simulink library "RadarImagingAndPositioning"  (R2018a)
settings: Solver=VariableStepAuto  StartTime=0.0  StopTime=10.0  RelTol=1e-3
undefined symbols (not defined in the file): fft2, gather, get, gpuArray, Time, us
libraries: dspobslib x8, dspstat3 x3, visionsinks x2, dspfdesign x2, commsdrhw_v2 x1, dspbuff3 x1, visiontransforms x1, dspsigops x1
settings Model: Creator=Sky  LastModifiedBy=Sky

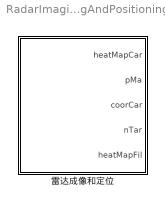
== system RadarImagingAndPositioning ==
  雷达成像和定位 : Subsystem  mask{yLoDownFac=2, nCyclePF=1, lFftAng=128, lFftDis=256, yMi=1, yMa=10, nTarMa=5, nFavr=40, pBackThres=0.0125, lWfil=3, pRelaThres=10, doSaveParam=on, decimInterp=100, rxBits=logical(dec2bin(0:11)-48), txBits=logical(dec2bin(0:3)-48), rxCoor=single([linspace(-0.053*(12/2-0.5),0.053*(12/2-0.5),12)',zeros(12,2)]), txCoor=single([zeros(4,2),linspace(-0.138-0.053*3,-0.138,4)']), dCa=4.65+0.5, fRamp=2000, fCen=3.2e9, fBw=1e9, tPul=0.0245e-3, tPulF=0.050e-3, trEdge=0, trThres=0}
      mask prompts: yLoDownFac "yLo downsample factor"; nCyclePF "cycles per frame (average time)"; lFftAng "angle FFT length"; lFftDis "dis FFT length"; yMi "y min"; yMa "y max"; nTarMa "targets number max"; nFavr "average frames"; pBackThres "background power threshold"; lWfil "filter window width"; pRelaThres "targets relative threshold"; doSaveParam "save parameters to workspace"; decimInterp "decimation factor"; rxBits "Rx bits"; txBits "Tx bits"; rxCoor "rx coordinates"; txCoor "tx coordinates"; dCa "cable length"; fRamp "ramp frequency"; fCen "center frequency"; fBw "bandwidth"; tPul "pulse width"; tPulF "first pulse width"; trEdge "triger edge"; trThres "triger threshold"
      mask help:
      | 雷达成像和定位模块。包含雷达成像和目标检测的主要算法。参数中USRP、Hardware、Ramp Parameters板块下的参数均与硬件有关，若有调整需求，请联系作者。
      |
      | 端口说明：
      | - heatMapCar：笛卡尔坐标系的雷达图像，经过对比度调整可以直接显示。
      | - pMa：雷达图像最大功率值。参考该值设置Targeting Parameters板块下的background power threshold参数，保证无人状态下的pMa小于参数background power threshold。算法原理：当pMa < background power threshold时判定区域内没有目标，此时端口nTar输出的值为0。
      | - coorTar：n行2列的矩阵，n个目标的坐标，单位（m）。第1列为x坐标，第2列为y坐标。前nTar个坐标为有效坐标。
      | - nTar：目标的个数。
      | - heatMapFil：滤波后的图像。算法原理：由于帧平均后的图像一个目标可能引起多个峰值，因此对图像进行一次以filter window width为正方形窗口宽度的中值滤波和均值滤波。增加filter window width使滤波后的图像更加平滑，减少一个目标检测到多个点的可能，同时会增加运算量。该端口用作参考以对filter window width进行修改。
      |
      | 参数说明：参数中Preprocess、FFT、Imaging、Targeting Parameters板块下的参数影响了运算量和目标检测效果。
      | - Preprocess Parameters：
      |     - yLo downsample factor：中频信号软件降采样系数。增大此值以减小运算量，同时减小距离测量范围。
      |     - cycles per frame（average time）：每帧包含的天线扫描周期。算法原理：将多个周期的中频信号平均，合并为一帧。增大此值以减小运算量，同时降低帧率。
      | - FFT Parameters：
      |     - angle FFT length：角度方向的FFT长度，设置为2的幂次方以使用更快的FFT算法。
      |     - dis FFT length：距离方向的FFT长度，设置为2的幂次方以使用更快的FFT算法。
      | - Imaging Parameters：
      |     - y min（max）：距离方向（y 方向）的坐标范围，直接影响雷达图像的行数和坐标序列ys，单位（m）。算法原理：两个参数会将2DFFT后的矩阵在距离方向（y方向）上作截取，如果dis FFT length参数设置的FFT长度达不到y max参数要求的FFT长度，会自动截取到dis FFT length所能计算到的最远距离，此ys表示的坐标序列不再以y max为最大值。
      | - Targeting Parameters：
      |     - target number max：最大跟踪目标数量。
      |     - average frames：滑动均值滤波的窗口宽度。算法原理：多径效应对成像造成的影响一般呈现出瞬时性，如果通过滑动均值滤波的方法平均多帧雷达图像，可以大大减弱多径效应的影响。同时均值滤波会带来与窗口长度相同的延迟。
      |     - background power threshold：背景功率阈值。参考pMa端口输出的功率设置Targeting Parameters板块下的background power threshold参数，保证无人状态下的pMa小于参数background power threshold。算法原理：当pMa < background power threshold时判定区域内没有目标，此时端口nTar输出的值为0。
      |     - filter window width：图像滤波的窗口宽度，设置为3以上的奇数（如3、5、7……）。算法原理：由于帧平均后的图像一个目标可能引起多个峰值，因此对图像进行一次以filter window width为正方形窗口宽度的中值滤波和均值滤波。增加此值使滤波后的图像更加平滑，减少一个目标检测到多个点的可能，同时会增加运算量。可以参考端口heaMapFil输出的滤波后的图像对该值进行修改。
      |     - targets relative threshold：目标功率相对与背景噪声功率比值的阈值。算法原理：以背景噪声平均值的targets relative threshold倍作为阈值对图像进行分割，高于此阈值的像素认为有目标存在。
      mask init:
      | if doSaveParam
      |     evalin('base','clear');
      | end
      | 
      | % 天线和斜坡参数
      | nRx=size(rxBits,1);
      | nTx=size(txBits,1);
      | lFraw=100e6/decimInterp/fRamp*nRx*nTx*nCyclePF;
      | fSraw=100e6/decimInterp;
      | fSdown=fSraw/yLoDownFac;
      | fF=fSraw/lFraw;
      | lRampRaw=fSraw/fRamp;%length ramp raw
      | lRampDown=lRampRaw/yLoDownFac;%length ramp downsample
      | nPul=size(rxBits,2)+size(txBits,2)+1;
      | lPul=fSraw*tPul;%length pulse
      | lPulF=fSraw*tPulF;%length pulse first
      | 
      | dLambda=3e8/fCen;
      | fPm=fBw*fRamp/3e8;%frequency per meter
      | fD=fSdown/lFftDis;%frequency delta
      | fs=single(linspace(0,fSraw/yLoDownFac/2-fD,floor(lFftDis/2)));
      | ds=fs/fPm;
      | 
      | angMax=asind(dLambda/2/abs(rxCoor(1,1)-rxCoor(2,1)));
      | angs=single(linspace(-angMax,angMax,lFftAng));
      | 
      | % 排除线缆长度，截取有效距离
      | dsVal=(ds(ds>=dCa)-dCa)/2;
      | isDval=single(find(dsVal>=yMi & dsVal<=yMa));
      | dsVal=dsVal(isDval);
      | isDval=isDval+find(ds>=dCa,1)-1;
      | 
      | % 一个斜坡内的时间
      | tsRampDown=single((0:lRampRaw/yLoDownFac-1)/fSraw*yLoDownFac);
      | isDown=yLoDownFac:yLoDownFac:lFraw;
      | 
      | % 极坐标转换后的xy坐标
      | ys=dsVal;
      | xsMax=sind(max(abs(angs)))*max(abs(dsVal));
      | xs=linspace(-xsMax,xsMax,length(angs));
      | [xss,yss]=meshgrid(xs,ys);
      | 
      | % 极坐标转换矩阵
      | dsPo2Car=sqrt(xss.^2+yss.^2);
      | angsPo2Car=atand(xss./yss);
      | angsPo2Car(isnan(angsPo2Car))=0;
      | 
      | % 计算衰减因子
      | facD=repmat((dsVal.^4)',1,length(angs));
      | 
      | % 保存参数到工作空间base
      | if doSaveParam
      |     % mask变量
      |     assignin('base','rxBits',rxBits);
      |     assignin('base','txBits',txBits);
      |     assignin('base','rxCoor',rxCoor);
      |     assignin('base','txCoor',txCoor);
      |     assignin('base','dCa',dCa);
      |     assignin('base','fRamp',fRamp);
      |     assignin('base','fCen',fCen);
      |     assignin('base','fBw',fBw);
      |     assignin('base','tPul',tPul);
      |     assignin('base','yLoDownFac',yLoDownFac);
      |     assignin('base','nCyclePF',nCyclePF);
      |     assignin('base','lFftAng',lFftAng);
      |     assignin('base','lFftDis',lFftDis);
      | 
      |     assignin('base','yMi',yMi);
      |     assignin('base','yMa',yMa);
      |     
      |     % 全局变量
      |     assignin('base','nRx',nRx);
      |     assignin('base','nTx',nTx);
      |     assignin('base','lFraw',lFraw);
      |     assignin('base','fF',fF);
      |     assignin('base','fSraw',fSraw);
      |     assignin('base','fSdown',fSdown);
      |     assignin('base','fPm',fPm);
      |     assignin('base','lRampRaw',lRampRaw);
      |     assignin('base','lRampDown',lRampDown);
      |     assignin('base','dLambda',dLambda);
      |     assignin('base','ds',ds);
      |     assignin('base','angs',angs);
      |     assignin('base','dsVal',dsVal);
      |     assignin('base','isDval',isDval);
      |     assignin('base','tsRamp',tsRampDown);
      |     assignin('base','xs',xs);
      |     assignin('base','ys',ys);
      |     assignin('base','xss',xss);
      |     assignin('base','yss',yss);
      |     assignin('base','facD',facD);
      | end
      mask TypeOptions decimInterp: SDRu Receiver/decimInterp
      mask DialogControl Container16 Prompt: 软件相关
      mask DialogControl preParams Prompt: Preprocess Parameters
      mask DialogControl fftParams Prompt: FFT Parameters
      mask DialogControl imagParams Prompt: Imaging Parameters
      mask DialogControl tarParams Prompt: Targeting Parameters
      mask DialogControl tabHardwareRelated Prompt: 硬件相关
      mask DialogControl simParam Prompt: sim parameters
      mask DialogControl USRPparams Prompt: USRP Parameters
      mask DialogControl hwParams Prompt: Hardware Parameters
      mask DialogControl rampParams Prompt: Ramp Parameters
      mask DialogControl tabDescription Prompt: 说明

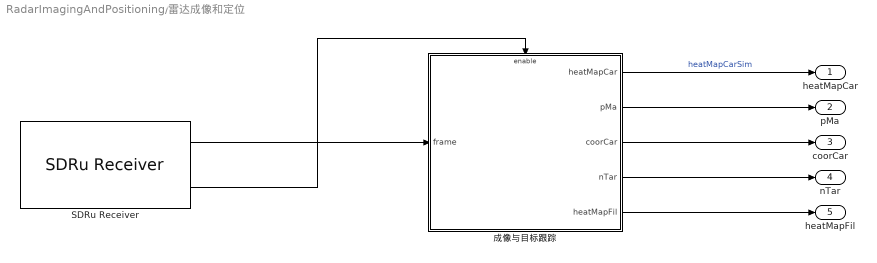
== system RadarImagingAndPositioning/雷达成像和定位 ==
  SDRu Receiver : commsdrhw_v2/SDRu Receiver  SourceLibraryInfo="This block requires <a href=\"http://www.mathworks.com/hardware-support/usrp.html\">Communications System Toolbox Support Package for USRP Radio</a>"  rxtx=rx  initializeIPAddress=0  devMap=0  USRP2_IP=192.168.10.6  USRP_IP_X300=192.168.10.2  USRP_IP_X310=192.168.10.2  USRP_serialNumB200=No devices found  USRP_serialNumB210=No devices found  platform=N200/N210/USRP2  prevPlatform=N200/N210/USRP2  lastIPAddressPopup=192.168.10.2  USRP_ID=192.168.10.6  LastIPAddress=192.168.10.2  ChannelMapping=1  centerFrequencySrc=Dialog  centerFrequency=0  loOffsetSrc=Dialog  loOffset=0  gainSrc=Dialog  gain=0  PPSSource=Internal  clockSource=Internal  masterClkRateParam=100e6  masterClkRateB200=32e6  masterClkRateB210=32e6  masterClkRateX300=200e6  masterClkRateX310=200e6  masterClkRate=100e6  decimInterpSrc=Dialog  decimInterp=decimInterp  USRP2_IP_NUM=[49 57 50 46 49 54 56 46 49 48 46 54]  TransportDataType=int16  overrunUnderrunPort=off  sampleTime=decimInterp/100e6  outputDatatype=single  frameLength=lFraw  HOST_DATA_PORT=0  HOST_CONTROL_PORT=0  USRP2_DATA_PORT=0  USRP2_CONTROL_PORT=0  bufferMode=Continuous streaming  EnableBurstMode=off  NumFramesInBurst=10000
      settings: SourceProductName=Communications System Toolbox Support Package for USRP(R) Radio  SourceProductBaseCode=USRP
  成像与目标跟踪 : Subsystem
  heatMapCar : Outport
  pMa : Outport  Port=2
  coorCar : Outport  Port=3
  nTar : Outport  Port=4
  heatMapFil : Outport  Port=5
  wires:
  SDRu Receiver/2 -> 成像与目标跟踪/Enable
  SDRu Receiver/1 -> 成像与目标跟踪/1(frame)
  成像与目标跟踪/1(heatMapCar) -> heatMapCar/1  "heatMapCarSim"
  成像与目标跟踪/4(nTar) -> nTar/1
  成像与目标跟踪/2(pMa) -> pMa/1
  成像与目标跟踪/3(coorCar) -> coorCar/1
  成像与目标跟踪/5(heatMapFil) -> heatMapFil/1

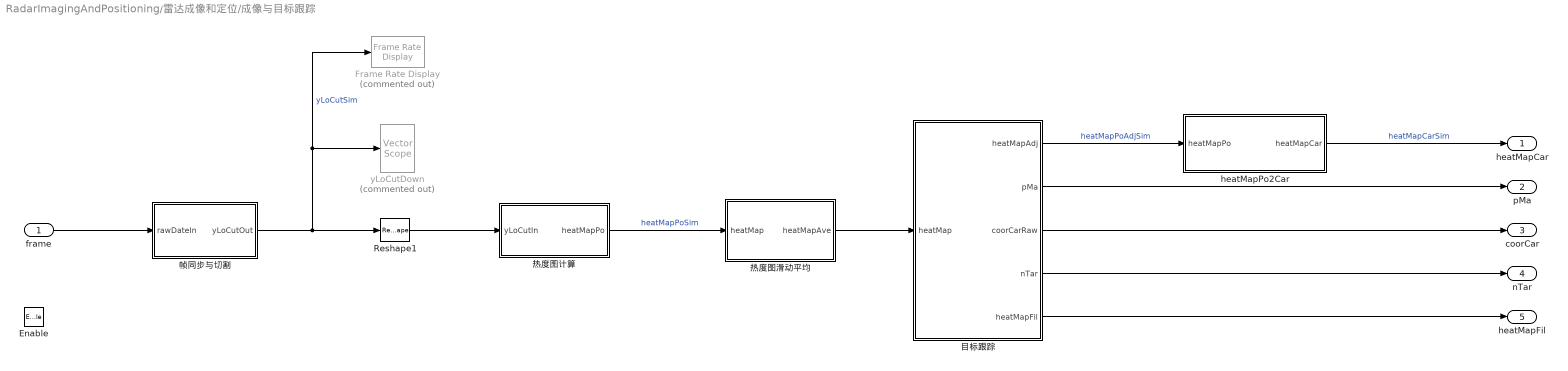
== system RadarImagingAndPositioning/雷达成像和定位/成像与目标跟踪 ==
  frame : Inport
  Enable : EnablePort  PropagateVarSize=During execution
  Frame Rate Display : visionsinks/Frame Rate Display  Commented=on  UpdateRate=10
      settings: SourceProductName=Computer Vision System Toolbox  SourceProductBaseCode=VP
  Reshape1 : Reshape  OutputDimensionality=Customize  OutputDimensions=[lRampDown,nRx,nTx]
  heatMapPo2Car : MATLAB Function  TreatAsAtomicUnit=on
  yLoCutDown : dspobslib/Vector Scope  Commented=on  ScopeProperties=on  Domain=User-defined  HorizSpan=1  DisplayProperties=off  AxisGrid=on  Memory=off  FrameNumber=on  AxisLegend=off  AxisZoom=off  OpenScopeAtSimStart=on  OpenScopeImmediately=off  FigPos=get(0,'defaultfigureposition')  AxisProperties=off  XUnits=Hertz  XRange=[0...Fs/2]  InheritXIncr=off  XIncr=1e6/fSdown  XLabel=Time(us)  XLimit=Auto  XMin=0  XMax=1  XStart=0  YUnits=dB  YLabel=Amplitude  LineProperties=off  LineColors=[1 0 0]|[0 1 0]|[0 0 1]  XAxisParamsVer=6.9
      settings: SourceProductName=DSP System Toolbox  SourceProductBaseCode=DS  YMin=-0.3  YMax=0.3
  帧同步与切割 : Subsystem
  热度图滑动平均 : Subsystem
  热度图计算 : Subsystem
  目标跟踪 : Subsystem
  heatMapCar : Outport
  pMa : Outport  Port=2
  coorCar : Outport  Port=3
  nTar : Outport  Port=4
  heatMapFil : Outport  Port=5
  wires:
  目标跟踪/1(heatMapAdj) -> heatMapPo2Car/1(heatMapPo)  "heatMapPoAdjSim"
  热度图滑动平均/1(heatMapAve) -> 目标跟踪/1(heatMap)
  热度图计算/1(heatMapPo) -> 热度图滑动平均/1(heatMap)  "heatMapPoSim"
  目标跟踪/3(coorCarRaw) -> coorCar/1
  帧同步与切割/1(yLoCutOut) -> Reshape1/1, Frame Rate Display/1, yLoCutDown/1  "yLoCutSim"
  frame/1 -> 帧同步与切割/1(rawDateIn)
  Reshape1/1 -> 热度图计算/1(yLoCutIn)
  目标跟踪/2(pMa) -> pMa/1
  目标跟踪/4(nTar) -> nTar/1
  heatMapPo2Car/1(heatMapCar) -> heatMapCar/1  "heatMapCarSim"
  目标跟踪/5(heatMapFil) -> heatMapFil/1

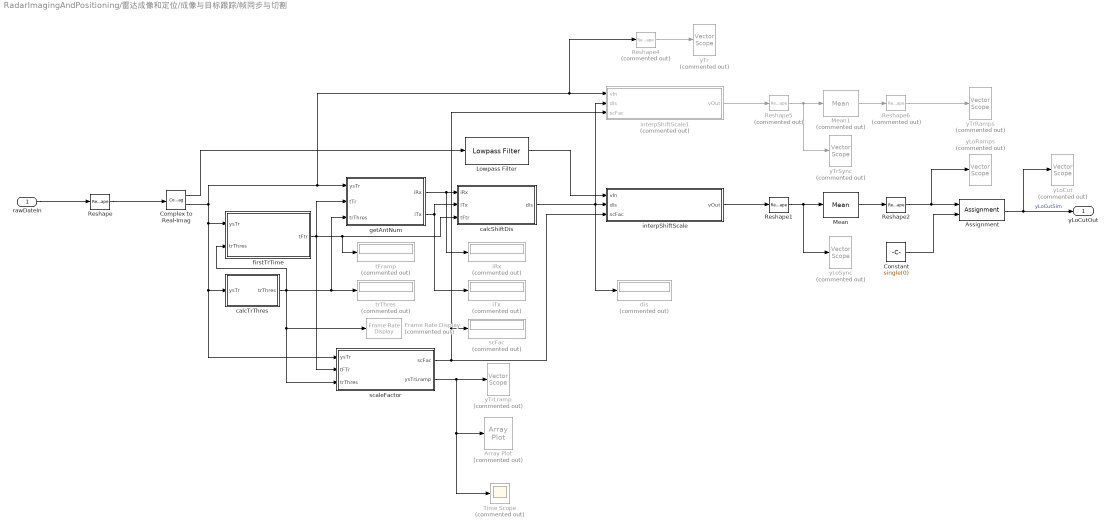
== system RadarImagingAndPositioning/雷达成像和定位/成像与目标跟踪/帧同步与切割 ==
  rawDateIn : Inport
  Array Plot : ArrayPlot  Commented=on
  Assignment : Assignment  NumberOfDimensions=2  DiagnosticForDimensions=Warning  IndexOptions=Index vector (dialog),Assign all  Indices=[1:ceil(2e-5*fSdown),lRampDown-ceil(2e-5*fSdown):lRampDown],1  OutputSizes=1,1
  Complex to Real-Imag : ComplexToRealImag
  Constant : Constant  Value=single(0)
  Frame Rate Display : visionsinks/Frame Rate Display  Commented=on  UpdateRate=10
      settings: SourceProductName=Computer Vision System Toolbox  SourceProductBaseCode=VP
  Lowpass Filter : dspfdesign/Lowpass Filter  FilterType=FIR  DesignForMinimumOrder=on  FilterOrder=20  PassbandFrequency=0.3*fSdown  StopbandFrequency=min(0.7*fSdown,0.5*fSraw)  PassbandRipple=0.1  StopbandAttenuation=50  InheritSampleRate=off  SampleRate=fSraw  SimulateUsing=Interpreted execution  roundingMode=Floor  coeffsDataTypeStr=fixdt(1,16)
  Mean : dspstat3/Mean  run=off  InputProcessing=Columns as channels (frame based)  reset_popup=None  directionMode=Each row  dimension=1  roiEnable=off  roiType=Rectangles  roiPortion=Entire ROI  roiOutput=Individual statistics for each ROI  roiFlag=off  roundingMode=Floor  overflowMode=off  outputDataTypeStr=Inherit: Same as accumulator  outputMin=[]  outputMax=[]  outputLastDataTypeStr=Inherit: Same as accumulator
  Mean1 : dspstat3/Mean  Commented=on  run=off  InputProcessing=Columns as channels (frame based)  reset_popup=None  directionMode=Each row  dimension=1  roiEnable=off  roiType=Rectangles  roiPortion=Entire ROI  roiOutput=Individual statistics for each ROI  roiFlag=off  roundingMode=Floor  overflowMode=off  outputDataTypeStr=Inherit: Same as accumulator  outputMin=[]  outputMax=[]  outputLastDataTypeStr=Inherit: Same as accumulator
  Reshape : Reshape  OutputDimensionality=Column vector (2-D)
  Reshape1 : Reshape  OutputDimensionality=Customize  OutputDimensions=[lRampDown*nRx*nTx,nCyclePF]
  Reshape2 : Reshape  OutputDimensionality=Customize  OutputDimensions=[lRampDown,nRx*nTx]
  Reshape4 : Reshape  Commented=on  OutputDimensionality=Column vector (2-D)
  Reshape5 : Reshape  Commented=on  OutputDimensionality=Customize  OutputDimensions=[lRampDown*nRx*nTx,nCyclePF]
  Reshape6 : Reshape  Commented=on  OutputDimensionality=Customize  OutputDimensions=[lRampDown,nRx*nTx]
  Time Scope : Scope  Commented=on
  calcShiftDis : MATLAB Function  TreatAsAtomicUnit=on
  calcTrThres : MATLAB Function  TreatAsAtomicUnit=on
  dis : Display  Commented=on
  firstTrTime : MATLAB Function  TreatAsAtomicUnit=on
  getAntNum : MATLAB Function  TreatAsAtomicUnit=on
  iRx : Display  Commented=on
  iTx : Display  Commented=on
  interpShiftScale : MATLAB Function  TreatAsAtomicUnit=on
  interpShiftScale1 : MATLAB Function  Commented=on  TreatAsAtomicUnit=on
  scFac : Display  Commented=on
  scaleFactor : MATLAB Function  TreatAsAtomicUnit=on
  tFramp : Display  Commented=on
  trThres : Display  Commented=on
  yLoCut : dspobslib/Vector Scope  Commented=on  ScopeProperties=on  Domain=User-defined  HorizSpan=1  DisplayProperties=off  AxisGrid=on  Memory=off  FrameNumber=on  AxisLegend=off  AxisZoom=off  OpenScopeAtSimStart=on  OpenScopeImmediately=off  FigPos=get(0,'defaultfigureposition')  AxisProperties=off  XUnits=Hertz  XRange=[0...Fs/2]  InheritXIncr=off  XIncr=1e6/fSdown  XLabel=Time(us)  XLimit=Auto  XMin=0  XMax=1  XStart=0  YUnits=dB  YLabel=Amplitude  LineProperties=off  LineColors=[1 0 0]|[0 1 0]|[0 0 1]  XAxisParamsVer=6.9
      settings: SourceProductName=DSP System Toolbox  SourceProductBaseCode=DS  YMin=-0.3  YMax=0.3
  yLoRamps : dspobslib/Vector Scope  Commented=on  ScopeProperties=on  Domain=User-defined  HorizSpan=1  DisplayProperties=off  AxisGrid=on  Memory=off  FrameNumber=on  AxisLegend=off  AxisZoom=off  OpenScopeAtSimStart=on  OpenScopeImmediately=off  FigPos=get(0,'defaultfigureposition')  AxisProperties=off  XUnits=Hertz  XRange=[0...Fs/2]  InheritXIncr=off  XIncr=1e6/fSdown  XLabel=Time(us)  XLimit=Auto  XMin=0  XMax=1  XStart=0  YUnits=dB  YLabel=Amplitude  LineProperties=off  LineColors=[1 0 0]|[0 1 0]|[0 0 1]  XAxisParamsVer=6.9
      settings: SourceProductName=DSP System Toolbox  SourceProductBaseCode=DS  YMin=-0.3  YMax=0.3
  yLoSync : dspobslib/Vector Scope  Commented=on  ScopeProperties=on  Domain=User-defined  HorizSpan=1  DisplayProperties=off  AxisGrid=on  Memory=off  FrameNumber=on  AxisLegend=off  AxisZoom=off  OpenScopeAtSimStart=on  OpenScopeImmediately=off  FigPos=get(0,'defaultfigureposition')  AxisProperties=off  XUnits=Hertz  XRange=[0...Fs/2]  InheritXIncr=off  XIncr=1e6/fSdown  XLabel=Time(us)  XLimit=Auto  XMin=0  XMax=1  XStart=0  YUnits=dB  YLabel=Amplitude  LineProperties=off  LineColors=[1 0 0]|[0 1 0]|[0 0 1]  XAxisParamsVer=6.9
      settings: SourceProductName=DSP System Toolbox  SourceProductBaseCode=DS  YMin=-0.3  YMax=0.3
  yTr : dspobslib/Vector Scope  Commented=on  ScopeProperties=on  Domain=User-defined  HorizSpan=1  DisplayProperties=off  AxisGrid=on  Memory=off  FrameNumber=on  AxisLegend=off  AxisZoom=off  OpenScopeAtSimStart=on  OpenScopeImmediately=off  FigPos=get(0,'defaultfigureposition')  AxisProperties=off  XUnits=Hertz  XRange=[0...Fs/2]  InheritXIncr=off  XIncr=1e6/fSraw  XLabel=Time(us)  XLimit=Auto  XMin=0  XMax=1  XStart=0  YUnits=dB  YLabel=Amplitude  LineProperties=off  LineColors=[1 0 0]|[0 1 0]|[0 0 1]  XAxisParamsVer=6.9
      settings: SourceProductName=DSP System Toolbox  SourceProductBaseCode=DS  YMin=-0.6  YMax=0.2
  yTrLramp : dspobslib/Vector Scope  Commented=on  ScopeProperties=on  Domain=User-defined  HorizSpan=1  DisplayProperties=off  AxisGrid=on  Memory=off  FrameNumber=on  AxisLegend=off  AxisZoom=off  OpenScopeAtSimStart=on  OpenScopeImmediately=off  FigPos=get(0,'defaultfigureposition')  AxisProperties=off  XUnits=Hertz  XRange=[0...Fs/2]  InheritXIncr=off  XIncr=1e6/fSraw  XLabel=Time(us)  XLimit=Auto  XMin=0  XMax=1  XStart=0  YUnits=dB  YLabel=Amplitude  LineProperties=off  LineColors=[1 0 0]|[0 1 0]|[0 0 1]  XAxisParamsVer=6.9
      settings: SourceProductName=DSP System Toolbox  SourceProductBaseCode=DS  YMin=-0.6  YMax=0.3
  yTrRamps : dspobslib/Vector Scope  Commented=on  ScopeProperties=on  Domain=User-defined  HorizSpan=1  DisplayProperties=off  AxisGrid=on  Memory=off  FrameNumber=on  AxisLegend=off  AxisZoom=off  OpenScopeAtSimStart=on  OpenScopeImmediately=off  FigPos=get(0,'defaultfigureposition')  AxisProperties=off  XUnits=Hertz  XRange=[0...Fs/2]  InheritXIncr=off  XIncr=1e6/fSdown  XLabel=Time(us)  XLimit=Auto  XMin=0  XMax=1  XStart=0  YUnits=dB  YLabel=Amplitude  LineProperties=off  LineColors=[1 0 0]|[0 1 0]|[0 0 1]  XAxisParamsVer=6.9
      settings: SourceProductName=DSP System Toolbox  SourceProductBaseCode=DS  YMin=-0.6  YMax=0.3
  yTrSync : dspobslib/Vector Scope  Commented=on  ScopeProperties=on  Domain=User-defined  HorizSpan=1  DisplayProperties=off  AxisGrid=on  Memory=off  FrameNumber=on  AxisLegend=off  AxisZoom=off  OpenScopeAtSimStart=on  OpenScopeImmediately=off  FigPos=get(0,'defaultfigureposition')  AxisProperties=off  XUnits=Hertz  XRange=[0...Fs/2]  InheritXIncr=off  XIncr=1e6/fSdown  XLabel=Time(us)  XLimit=Auto  XMin=0  XMax=1  XStart=0  YUnits=dB  YLabel=Amplitude  LineProperties=off  LineColors=[1 0 0]|[0 1 0]|[0 0 1]  XAxisParamsVer=6.9
      settings: SourceProductName=DSP System Toolbox  SourceProductBaseCode=DS  YMin=-0.6  YMax=0.3
  yLoCutOut : Outport
  wires:
  firstTrTime/1(tFtr) -> scaleFactor/2(tFTr), getAntNum/2(tTr), tFramp/1, calcShiftDis/3(tFtr)
  getAntNum/1(iRx) -> iRx/1, calcShiftDis/1(iRx)
  Complex to Real-Imag/1 -> Lowpass Filter/1
  Reshape/1 -> Complex to Real-Imag/1
  interpShiftScale/1(vOut) -> Reshape1/1
  Reshape2/1 -> yLoRamps/1, Assignment/1
  calcTrThres/1(trThres) -> firstTrTime/2(trThres), scaleFactor/3(trThres), Frame Rate Display/1, trThres/1, getAntNum/3(trThres)
  Constant/1 -> Assignment/2
  calcShiftDis/1(dis) -> interpShiftScale1/2(dis), dis/1, interpShiftScale/2(dis)
  Mean/1 -> Reshape2/1
  rawDateIn/1 -> Reshape/1
  Assignment/1 -> yLoCutOut/1, yLoCut/1  "yLoCutSim"
  Reshape4/1 -> yTr/1
  Reshape1/1 -> yLoSync/1, Mean/1
  getAntNum/2(iTx) -> iTx/1, calcShiftDis/2(iTx)
  scaleFactor/2(ysTrLramp) -> Time Scope/1, Array Plot/1, yTrLramp/1
  interpShiftScale1/1(vOut) -> Reshape5/1
  Mean1/1 -> Reshape6/1
  Reshape5/1 -> yTrSync/1, Mean1/1
  Reshape6/1 -> yTrRamps/1
  scaleFactor/1(scFac) -> interpShiftScale1/3(scFac), scFac/1, interpShiftScale/3(scFac)
  Lowpass Filter/1 -> interpShiftScale/1(vIn)
  Complex to Real-Imag/2 -> scaleFactor/1(ysTr), calcTrThres/1(ysTr), firstTrTime/1(ysTr), interpShiftScale1/1(vIn), Reshape4/1, getAntNum/1(ysTr)

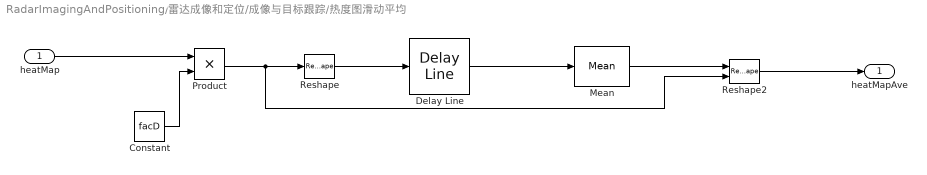
== system RadarImagingAndPositioning/雷达成像和定位/成像与目标跟踪/热度图滑动平均 ==
  heatMap : Inport
  Constant : Constant  Value=facD  VectorParams1D=off
  Delay Line : dspbuff3/Delay Line  siz=nFavr  ic=0  directfeed=off  enable_output=off  hold_output=off  OutputFrames=off
      settings: SourceProductName=DSP System Toolbox  SourceProductBaseCode=DS
  Mean : dspstat3/Mean  run=off  InputProcessing=Columns as channels (frame based)  reset_popup=None  directionMode=Specified dimension  dimension=1  roiEnable=off  roiType=Rectangles  roiPortion=Entire ROI  roiOutput=Individual statistics for each ROI  roiFlag=off  roundingMode=Floor  overflowMode=off  outputDataTypeStr=Inherit: Same as accumulator  outputMin=[]  outputMax=[]  outputLastDataTypeStr=Inherit: Same as accumulator
  Product : Product
  Reshape : Reshape  OutputDimensionality=Row vector (2-D)
  Reshape2 : Reshape  OutputDimensionality=Derive from reference input port
  heatMapAve : Outport
  wires:
  Delay Line/1 -> Mean/1
  Constant/1 -> Product/2
  Reshape2/1 -> heatMapAve/1
  Product/1 -> Reshape/1, Reshape2/2
  Mean/1 -> Reshape2/1
  Reshape/1 -> Delay Line/1
  heatMap/1 -> Product/1

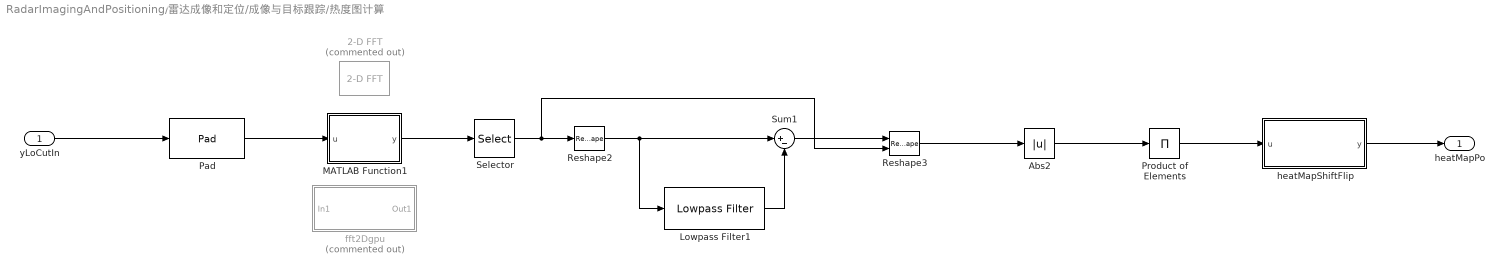
== system RadarImagingAndPositioning/雷达成像和定位/成像与目标跟踪/热度图计算 ==
  yLoCutIn : Inport
  2-D FFT : visiontransforms/2-D FFT  Commented=on  TableOpt=NEW  TableOptActive=Speed  BitRevOrder=off  SkipNorm=off  FFTImplementation=Auto  firstCoeffDataTypeStr=Inherit: Same word length as input  firstCoeffLastDataTypeStr=Inherit: Same word length as input  outputMin=[]  outputMax=[]  roundingMode=Floor  overflowMode=off
      settings: SourceProductName=Computer Vision System Toolbox  SourceProductBaseCode=VP
  Abs2 : Abs
  Lowpass Filter1 : dspfdesign/Lowpass Filter  FilterType=IIR  DesignForMinimumOrder=off  FilterOrder=1  PassbandFrequency=0.1  StopbandFrequency=3  PassbandRipple=0.1  StopbandAttenuation=30  InheritSampleRate=off  SampleRate=fF  SimulateUsing=Interpreted execution  roundingMode=Floor  coeffsDataTypeStr=fixdt(1,16)
  MATLAB Function1 : MATLAB Function  TreatAsAtomicUnit=on
  Pad : dspsigops/Pad  padAlong=Columns and rows  dimsToPad=1  valSrc=Specify via dialog  padVal=0  spec=Output size  padNumOutRowsSpecMethod=User-specified  numOutRows=lFftDis  padNumOutColsSpecMethod=User-specified  numOutCols=lFftAng  isVarDimsMode=off  padBeginning=0  padEnd=0  outSizeMode=User-specified  outSize=1  padSigAt=End  trunc_flag=None  roundingMode=Floor  overflowMode=off  truncOrWrapMode=Truncate  wrap_flag=None
      settings: SourceProductName=DSP System Toolbox  SourceProductBaseCode=DS
  Product of Elements : Product  Inputs=*  CollapseMode=Specified dimension  CollapseDim=3  OutDataTypeStr=Inherit: Same as first input
  Reshape2 : Reshape  OutputDimensionality=Row vector (2-D)
  Reshape3 : Reshape  OutputDimensionality=Derive from reference input port
  Selector : Selector  NumberOfDimensions=3  InputPortWidth=3  IndexOptions=Index vector (dialog),Select all,Select all  Indices=isDval,1,1  OutputSizes=1,1,1
  Sum1 : Sum  Inputs=|+-
  fft2Dgpu : Subsystem  Commented=on  TreatAsAtomicUnit=on
  heatMapShiftFlip : MATLAB Function  TreatAsAtomicUnit=on
  heatMapPo : Outport
  wires:
  Pad/1 -> MATLAB Function1/1(u)
  MATLAB Function1/1(y) -> Selector/1
  Lowpass Filter1/1 -> Sum1/2
  Abs2/1 -> Product of Elements/1
  Reshape2/1 -> Lowpass Filter1/1, Sum1/1
  yLoCutIn/1 -> Pad/1
  Product of Elements/1 -> heatMapShiftFlip/1(u)
  Selector/1 -> Reshape3/2, Reshape2/1
  Sum1/1 -> Reshape3/1
  Reshape3/1 -> Abs2/1
  heatMapShiftFlip/1(y) -> heatMapPo/1

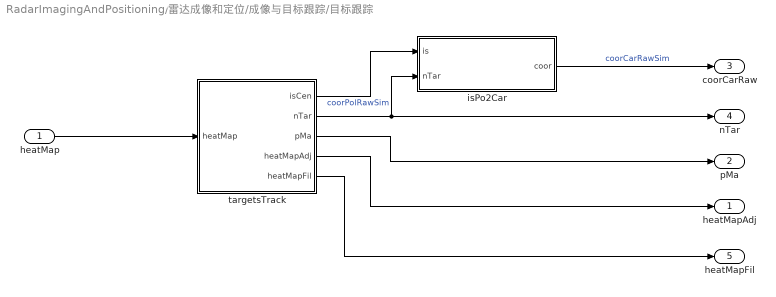
== system RadarImagingAndPositioning/雷达成像和定位/成像与目标跟踪/目标跟踪 ==
  heatMap : Inport
  isPo2Car : MATLAB Function  TreatAsAtomicUnit=on
  targetsTrack : MATLAB Function  TreatAsAtomicUnit=on
  heatMapAdj : Outport
  pMa : Outport  Port=2
  coorCarRaw : Outport  Port=3
  nTar : Outport  Port=4
  heatMapFil : Outport  Port=5
  wires:
  isPo2Car/1(coor) -> coorCarRaw/1  "coorCarRawSim"
  targetsTrack/1(isCen) -> isPo2Car/1(is)  "coorPolRawSim"
  heatMap/1 -> targetsTrack/1(heatMap)
  targetsTrack/2(nTar) -> isPo2Car/2(nTar), nTar/1
  targetsTrack/3(pMa) -> pMa/1
  targetsTrack/4(heatMapAdj) -> heatMapAdj/1
  targetsTrack/5(heatMapFil) -> heatMapFil/1

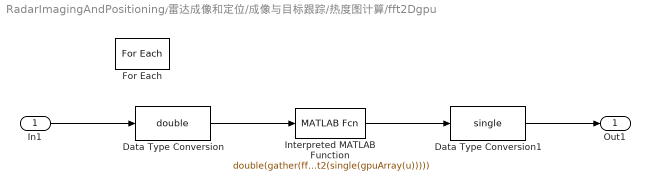
== system RadarImagingAndPositioning/雷达成像和定位/成像与目标跟踪/热度图计算/fft2Dgpu ==
  In1 : Inport  Partition=on  PartitionDimension=3  PartitionWidth=1  PartitionOffset=0
  Data Type Conversion : DataTypeConversion  OutDataTypeStr=double
  Data Type Conversion1 : DataTypeConversion  OutDataTypeStr=single
  For Each : ForEach  DisableCoverage=on  IndexMode=One-based
  Interpreted MATLAB Function : MATLABFcn  MATLABFcn=double(gather(fft2(single(gpuArray(u)))))  Output1D=off
  Out1 : Outport  ConcatenationDimension=3
  wires:
  In1/1 -> Data Type Conversion/1
  Interpreted MATLAB Function/1 -> Data Type Conversion1/1
  Data Type Conversion/1 -> Interpreted MATLAB Function/1
  Data Type Conversion1/1 -> Out1/1

== matlab function RadarImagingAndPositioning/雷达成像和定位/成像与目标跟踪/帧同步与切割/getAntNum ==
  data: ysTr input; tTr input; trThres input; iRx output; fSraw parameter; lPul parameter; nPul parameter; rxBits parameter; txBits parameter; iTx output; nTx parameter; nRx parameter; lPulF parameter
%% 判断触发时间对应同步信号的天线编号
% iRx: 接收天线编号
% iTx: 发射天线编号
% ysTr: 一帧triger信号
% tRamp: 斜坡开始时间，以第一个采样点为参考时间0
% fSraw: 原始采样率
% lPul: 一个脉冲/比特采样点数
% nPul: 脉冲/比特总数
% rxBits: 接收天线比特
% txBits: 发射天线比特
% trThres: 触发电平
% nRx: 接收天线数量
% nTx: 发射天线数量
function [iRx,iTx]=getAntNum(ysTr, tTr, trThres, fSraw, lPul, nPul, rxBits, txBits, nTx, nRx, lPulF)
if isnan(tTr)
    iRx=nan;
    iTx=nan;
    return
end
%% 准备参数
nPulRx=size(rxBits,2);
nPulTx=size(txBits,2);

%% 抽取天线编号的比特电平
iBit1=ceil(tTr*fSraw+lPulF+0.5*lPul)+1;

tsBits=round(linspace(iBit1,iBit1+lPul*(nPulRx+nPulTx-1),nPul-1));
isBits=mod(tsBits-1,length(ysTr))+1;
ysBits=ysTr(isBits)>trThres;
isRx=find(all(~xor(rxBits,repmat(ysBits(1:nPulRx)',nRx,1)),2),1);
isTx=find(all(~xor(txBits,repmat(ysBits(nPulRx+1:nPul-1)',nTx,1)),2),1);
if isempty(isRx)
    iRx=nan;
else
    iRx=isRx(1);%为simulink推理iRx大小提供帮助
end
if isempty(isTx)
    iTx=nan;
else
    iTx=isTx(1);%为simulink推理iTx大小提供帮助
end


end

== matlab function RadarImagingAndPositioning/雷达成像和定位/成像与目标跟踪/帧同步与切割/firstTrTime ==
  data: ysTr input; tFtr output; fSraw parameter; lRampRaw parameter; lPul parameter; nPul parameter; trEdge parameter; trThres input; nRx parameter; nTx parameter; nCyclePF parameter; lPulF parameter
%% 同步斜坡信号起始时间函数，返回所有斜坡信号起始时间点
% tFramp: 第一个斜坡开始时间，精确到采样时间之下，以第一个采样点为参考时间0
% ysTr: 一帧triger信号
% fSraw: 原始采样率
% lRampRaw: 一个斜坡的原始采样点数
% lPul: 一个脉冲/比特采样点数
% nPul: 脉冲/比特总数
% trEdge: 触发沿：1上升沿 0下降沿
% trThres: 触发电平
% nRx: 接收天线数量
% nTx: 发射天线数量
% nCyclePF: 每帧包含的天线扫描周期数
function tFtr=firstTrTime(ysTr, fSraw, lRampRaw, lPul, nPul, trEdge, trThres, nRx, nTx, nCyclePF, lPulF)

if(mod(length(ysTr),lRampRaw)~=0)
    error('The length of frame is not integer multiple of the length of ramp .');
end

%% 分析第一个完整斜坡同步信号
%第一个完整斜坡同步信号触发沿位于1:lRamp,为了容错，扩大范围到1:lRamp+lPul*nPul
lPulAll=lPulF+(lPul*nPul-1);
if(nRx*nTx*nCyclePF>1)
    isFramp=1:lRampRaw+lPulAll;%indexs first ramp
else
    isFramp=1:lRampRaw;
end
ysTrFf=ysTr(isFramp);%ys triger first ramp
isTr=[];
if trEdge==0
    isTr=find(ysTrFf(2:end)<trThres & ysTrFf(1:end-1)>=trThres)+1;%index triger first
else
    isTr=find(ysTrFf(2:end)>trThres & ysTrFf(1:end-1)<=trThres)+1;
end
iTrF=0;
if isempty(isTr)
    tFtr=nan;
    return
else
    iTrF=isTr(find([true,diff(isTr,1,1)'>lPulAll],1,'last'));%要求脉冲和比特总时长小于斜坡周期的一半,选取最后一个触发信号
end


%% 线性插值分析触发沿的精确时间
tFtr=interp1(double([ysTr(iTrF-1),ysTr(iTrF)]),double([iTrF-1,iTrF]-1)/fSraw,double(trThres));
end

== matlab function RadarImagingAndPositioning/雷达成像和定位/成像与目标跟踪/帧同步与切割/interpShiftScale1 ==
  data: vIn input; vOut output; dis input; scFac input; isDown parameter
%% 循环移位，通过线性插值实现小数位数的移位
% vOut: 输出向量
% vIn: 输入向量
% dis: 向右移位距离
function vOut=interpShiftScaleDownsample(vIn, dis, scFac, isDown)
    if isnan(dis)||isnan(scFac)
        vOut=vIn(isDown);
        return
    end
    isZeroBased=(0:length(vIn)-1)';
    dis=dis/scFac;
    if dis>=0
        iShift=floor(dis);
        iAdd=dis-iShift;
    else
        iShift=ceil(dis);
        iAdd=iShift-dis;
    end
    
    isShifted=circshift(isZeroBased,iShift);

    vOut=interp1(isZeroBased/scFac,vIn, ...
        isShifted(isDown)+iAdd,'linear','extrap');
end

== matlab function RadarImagingAndPositioning/雷达成像和定位/成像与目标跟踪/帧同步与切割/calcShiftDis ==
  data: iRx input; iTx input; dis output; tFtr input; lRampRaw parameter; fSraw parameter; nRx parameter; nTx parameter
%% 通过天线序号、时间偏移计算循环移位位移量
% dis: 位移量
% iAnt: 天线序号，从1开始
% tFtr: 第一个触发信号时间
% lRampRaw: 一个斜坡的原始采样点数
% fSraw: 原始采样率
% nRx: 接收天线数量
% nTx: 发射天线数量
function dis=calcShiftDis(iRx, iTx, tFtr, lRampRaw, fSraw, nRx, nTx)
    dis=-((nRx*nTx+1+nRx-iRx-nRx*iTx)*lRampRaw+(tFtr*fSraw));
end

== matlab function RadarImagingAndPositioning/雷达成像和定位/成像与目标跟踪/目标跟踪/isPo2Car ==
  data: is input; coor output; dsVal parameter; angs parameter; nTar input
function coor = isPo2Car(is, dsVal, angs, nTar)
coor=zeros(size(is),'single');
d=interp1(1:length(dsVal),dsVal,(is(1:nTar,2)));
ang=interp1(1:length(angs),angs,(is(1:nTar,1)));
coor(1:nTar,1)=d.*sind(ang);
coor(1:nTar,2)=d.*cosd(ang);

== matlab function RadarImagingAndPositioning/雷达成像和定位/成像与目标跟踪/帧同步与切割/calcTrThres ==
  data: ysTr input; trThres output
%% 计算触发电平
function trThres = calcTrThres(ysTr)
trThres=(max(ysTr)+min(ysTr))/2;%triger threshold
% trThres=(mean(ysTr(ysTr>trThres))+mean(ysTr(ysTr<trThres)))/2;
end

== matlab function RadarImagingAndPositioning/雷达成像和定位/成像与目标跟踪/热度图计算/MATLAB Function1 ==
  data: u input; y output
function y = fft2d(u)
y=fft2(u);

== matlab function RadarImagingAndPositioning/雷达成像和定位/成像与目标跟踪/热度图计算/heatMapShiftFlip ==
  data: u input; y output
function y = heatMapShiftFlip(u)
y =circshift(u,ceil(size(u,2)/2),2);
y=flip(y,2);

== matlab function RadarImagingAndPositioning/雷达成像和定位/成像与目标跟踪/帧同步与切割/scaleFactor ==
  data: ysTr input; tFTr input; trThres input; scFac output; fSraw parameter; fRamp parameter; trEdge parameter; nRx parameter; nTx parameter; nCyclePF parameter; ysTrLramp output
%% 同步斜坡信号起始时间函数，返回所有斜坡信号起始时间点
% scFac: 缩放因子，adf4159的时钟比usrp的时钟
% ysTrLramp: 输出最后一个触发沿的时域信号
% ysTr: 一帧triger信号
% tRamp: 斜坡开始时间，以第一个采样点为参考时间0
% trThres: 触发电平
% fSraw: 原始采样率
% fRamp: 斜坡频率
% trEdge: 触发沿：1上升沿 0下降沿
% nRx: 接收天线数量
% nTx: 发射天线数量
% nCyclePF: 每帧包含的天线扫描周期数
function [scFac, ysTrLramp]=scaleFactor(ysTr, tFTr, trThres, fSraw, fRamp, trEdge ,nRx, nTx, nCyclePF)
%% 准备参数
hW=ceil(nRx*nTx*nCyclePF*0.1);%half width

% 如果一个帧包含的ramp数小于3
% 可能导致无法定位最后一个ramp起始时间
% 因为tFramp可能识别为第一或二个ramp的起始时间
if isnan(tFTr) || nRx*nTx*nCyclePF<3
    scFac=nan;
    ysTrLramp=zeros(hW*2+1,1,'single');
    return
end

%% 根据第一个斜坡开始时间（tFramp）计算最后一个斜坡开始时间区间
iCen=round(tFTr*fSraw+fSraw/fRamp*(nRx*nTx*nCyclePF-2));
isLramp=(-hW:hW)+iCen;
ysTrLramp=ysTr(isLramp);

%% 分析最后一个斜坡开始时间
if trEdge==0
    isTr=find(ysTrLramp(2:end)<trThres & ysTrLramp(1:end-1)>=trThres)+1;%index triger first
else
    isTr=find(ysTrLramp(2:end)>trThres & ysTrLramp(1:end-1)<=trThres)+1;
end
iTrF=0;
if isempty(isTr)
    scFac=nan;
    ysTrLramp=zeros(hW*2+1,1,'single');
    return
else
    iTrF=isTr(1);
end

%% 线性插值分析触发沿的精确时间
tLramp=interp1(double([ysTrLramp(iTrF-1),ysTrLramp(iTrF)]),double([isLramp(iTrF)-1,isLramp(iTrF)]-1)/fSraw,double(trThres));
scFac=(tLramp-tFTr)*fRamp/(nRx*nTx*nCyclePF-2);
end

== matlab function RadarImagingAndPositioning/雷达成像和定位/成像与目标跟踪/目标跟踪/targetsTrack ==
  data: heatMap input; isCen output; nTar output; nTarMa parameter; pBackThres parameter; pMa output; heatMapAdj output; pRelaThres parameter; heatMapFil output; lWfil parameter
function [isCen,nTar,pMa,heatMapAdj,heatMapFil] = targetsTrack(heatMap, nTarMa, pBackThres, pRelaThres,lWfil)
isCen=zeros(nTarMa,2,'single');
pMa=max(heatMap(:));
if pMa<pBackThres
    nTar=single(0);
    heatMapAdj=heatMap/pBackThres;
    heatMapFil=heatMapAdj;
    return;
else
    heatMap(heatMap<pBackThres)=pBackThres;
    heatMapAdj=(heatMap-pBackThres)/(pMa-pBackThres);
    heatMapFil=heatMapAdj;
    
    heatMapFil = medfilt2(heatMapFil,[lWfil,lWfil]);
    heatMapFil=filter2(fspecial('average',[lWfil,lWfil]),heatMapFil);
    % pre = wiener2(pre,[5 13]);
    % se = strel('disk',3);
    % pre = imopen(pre,se);
    
    bw = imbinarize(heatMapFil,pRelaThres*mean(heatMapFil(:)));
    stats = regionprops(bw,double(heatMap),'Area','WeightedCentroid');
    
    nTar=min(single(length(stats)),nTarMa);
    for i=1:min(length(stats),nTarMa)
        isCen(i,:)=single(stats(i).WeightedCentroid);
    end
end

== matlab function RadarImagingAndPositioning/雷达成像和定位/成像与目标跟踪/帧同步与切割/interpShiftScale ==
  data: vIn input; vOut output; dis input; scFac input; isDown parameter
%% 循环移位，通过线性插值实现小数位数的移位
% vOut: 输出向量
% vIn: 输入向量
% dis: 向右移位距离
function vOut=interpShiftScaleDownsample(vIn, dis, scFac, isDown)
    if isnan(dis)||isnan(scFac)
        vOut=vIn(isDown);
        return
    end
    isZeroBased=(0:length(vIn)-1)';
    dis=dis/scFac;
    if dis>=0
        iShift=floor(dis);
        iAdd=dis-iShift;
    else
        iShift=ceil(dis);
        iAdd=iShift-dis;
    end
    
    isShifted=circshift(isZeroBased,iShift);

    vOut=interp1(isZeroBased/scFac,vIn, ...
        isShifted(isDown)+iAdd,'linear','extrap');
end

== matlab function RadarImagingAndPositioning/雷达成像和定位/成像与目标跟踪/heatMapPo2Car ==
  data: heatMapPo input; heatMapCar output; angs parameter; dsVal parameter; angsPo2Car parameter; dsPo2Car parameter
function heatMapCar = heatMapPo2Car(heatMapPo,angs, dsVal, angsPo2Car, dsPo2Car)
heatMapCar=interp2(angs,dsVal,heatMapPo,angsPo2Car,dsPo2Car,'linear',0);
